simulink model "fz5_2"  (R2014a)
settings: Solver=ode45  StartTime=0.0  StopTime=10.0  MaxStep=0.001  RelTol=1e-3
undefined symbols (not defined in the file or in its folder): magnitude
libraries: commanapbnd3 x1, dspstat3 x1, commrandsrc2 x1
settings Model: Creator=tzb  LastModifiedBy=tzb
settings DebuggingCC: SolverPrmCheckMsg=none

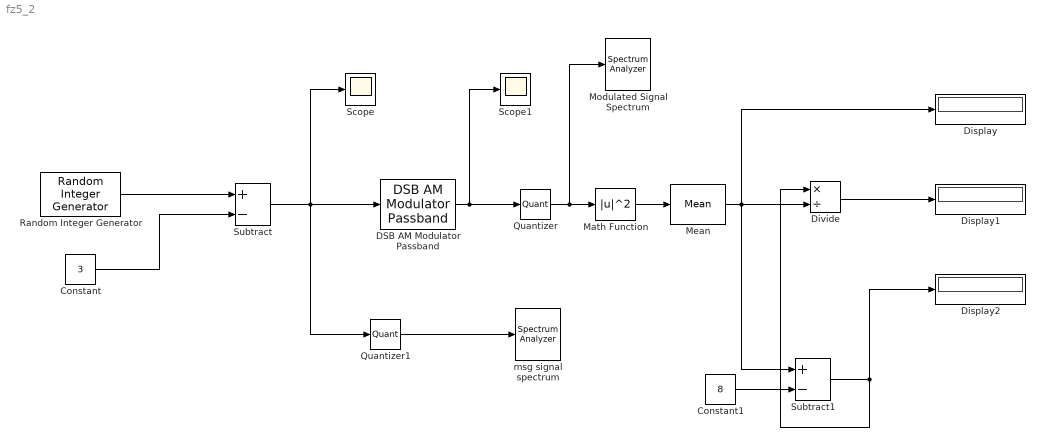
== system fz5_2 ==
  Constant : Constant  Value=3
  Constant1 : Constant  Value=8
  DSB AM Modulator Passband : commanapbnd3/DSB AM Modulator Passband  Fc=300  Ph=0  Offset=4
  Display : Display
  Display1 : Display
  Display2 : Display
  Divide : Product  Inputs=*/
  Math Function : Math  Operator=magnitude^2  SaturateOnIntegerOverflow=on
  Mean : dspstat3/Mean  run=on  reset_popup=None  InputProcessing=Columns as channels (frame based)  directionMode=Each column  dimension=1  treatSBRowAsCol=on  roiEnable=off  roiType=Rectangles  roiPortion=Entire ROI  roiOutput=Individual statistics for each ROI  roiFlag=off  outputDataTypeStr=Inherit: Same as accumulator  outputLastDataTypeStr=Inherit: Same as accumulator  outputMin=[]  outputMax=[]  roundingMode=Floor  overflowMode=off
  Modulated Signal Spectrum : SpectrumAnalyzer
  Quantizer : Quantizer  QuantizationInterval=0.001  SampleTime=0.001
  Quantizer1 : Quantizer  QuantizationInterval=0.001  SampleTime=0.001
  Random Integer Generator : commrandsrc2/Random Integer Generator  mul=7  seed=1234  Ts=1/10  frameBased=off  sampPerFrame=1  orient=off  outDataType=double
  Scope : Scope
  Scope1 : Scope
  Subtract : Sum  Inputs=+-
  Subtract1 : Sum  Inputs=+-
  msg signal spectrum : SpectrumAnalyzer
  wires:
  Random Integer Generator/1 -> Subtract/1
  Constant/1 -> Subtract/2
  Subtract/1 -> Quantizer1/1, Scope/1, DSB AM Modulator Passband/1
  Quantizer1/1 -> msg signal spectrum/1
  DSB AM Modulator Passband/1 -> Quantizer/1, Scope1/1
  Math Function/1 -> Mean/1
  Quantizer/1 -> Modulated Signal Spectrum/1, Math Function/1
  Constant1/1 -> Subtract1/2
  Mean/1 -> Display/1, Subtract1/1, Divide/2
  Divide/1 -> Display1/1
  Subtract1/1 -> Display2/1, Divide/1
